simulink model "ModelEnv_Test2"  (R2020b)
settings: Solver=VariableStepAuto  StartTime=0.0  StopTime=10  RelTol=1e-3
values from neighbouring files (symbols this model uses):
  Atz = -0.15    [AgentSaboteur.m]    (also in Test1_code.m; TesterUnAgent.m; test_RL_code.m; test_RL_code_v2.m)
  Bd = 0.03    [AgentSaboteur.m]    (also in Test1_code.m; TesterUnAgent.m; test_RL_code.m; test_RL_code_v2.m)
  Bh = mdot/(3*M)    (= 0.164794600011)    [AgentSaboteur.m]    (also in Test1_code.m; TesterUnAgent.m; test_RL_code.m; test_RL_code_v2.m)
  Tout = [7 6 5 6 4 4 6 8 9 10 11 12 14 14 16 17 14 12 10 9 8 8 7 6]    [AgentSaboteur.m]    (also in Test1_code.m = out.simout.Data(:, 1); Tout(end)=[]; TesterUnAgent.m; testBlanc.m = 13 + 2*rand(1, 240); test_RL_code.m)
  Tz_init = Tout(1)    [AgentSaboteur.m]    (also in Test1_code.m; TesterUnAgent.m; testBlanc.m; test_RL_code.m)
libraries: dspsrcs4 x1
settings Model: Creator=masdoua1  LastModifiedBy=masdoua1
settings SolverCC: AlgebraicLoopSolver=LineSearch

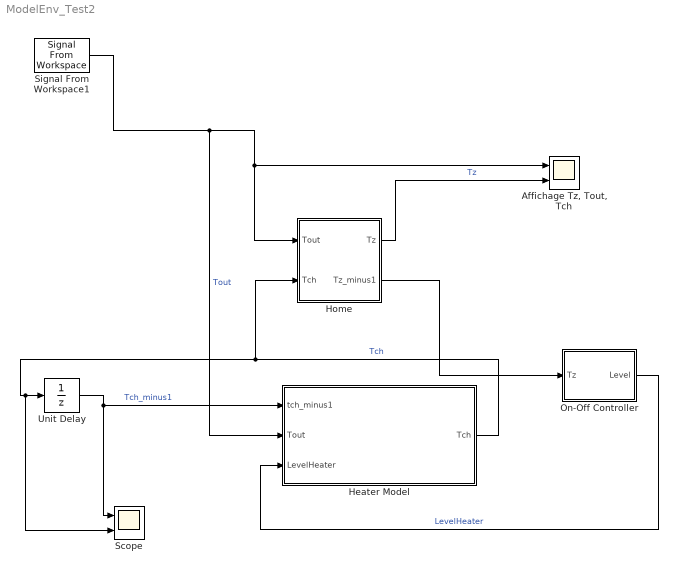
== system ModelEnv_Test2 ==
  "Affichage Tz, Tout, Tch" : Scope  NumInputPorts=2
  Heater Model : Subsystem
  Home : Subsystem
  On-Off Controller : MATLAB Function  TreatAsAtomicUnit=on
  Scope : Scope  NumInputPorts=2
  Signal From Workspace1 : dspsrcs4/Signal From Workspace  X=Tout  Ts=1  nsamps=1  OutputAfterFinalValue=Setting to zero  ignoreOrWarnInputAndFrameLengths=off  OutputFrames=off
  Unit Delay : UnitDelay  InitialCondition=Tout(1)  HasFrameUpgradeWarning=on
  wires:
  Signal From Workspace1/1 -> Heater Model/2(Tout), Home/1(Tout), "Affichage Tz, Tout, Tch"/1  "Tout"
  Home/1(Tz) -> "Affichage Tz, Tout, Tch"/2  "Tz"
  Heater Model/1(Tch) -> Scope/2, Unit Delay/1, Home/2(Tch)  "Tch"
  Unit Delay/1 -> Scope/1, Heater Model/1(tch_minus1)  "Tch_minus1"
  On-Off Controller/1(Level) -> Heater Model/3(LevelHeater)  "LevelHeater"
  Home/2(Tz_minus1) -> On-Off Controller/1(Tz)

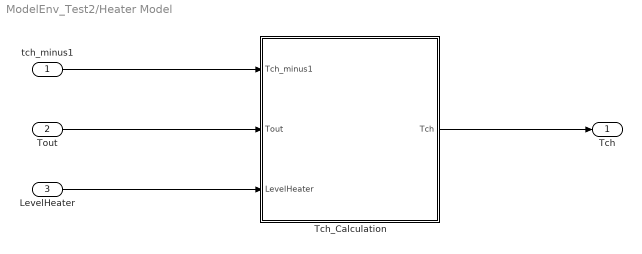
== system ModelEnv_Test2/Heater Model ==
  tch_minus1 : Inport
  Tout : Inport  Port=2
  LevelHeater : Inport  Port=3
  Tch_Calculation : MATLAB Function  TreatAsAtomicUnit=on
  Tch : Outport
  wires:
  Tout/1 -> Tch_Calculation/2(Tout)
  tch_minus1/1 -> Tch_Calculation/1(Tch_minus1)
  LevelHeater/1 -> Tch_Calculation/3(LevelHeater)
  Tch_Calculation/1(Tch) -> Tch/1

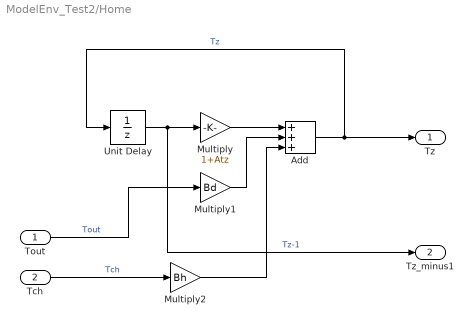
== system ModelEnv_Test2/Home ==
  Tout : Inport
  Tch : Inport  Port=2
  Add : Sum  Inputs=+++
  Multiply : Gain  Gain=1+Atz
  Multiply1 : Gain  Gain=Bd
  Multiply2 : Gain  Gain=Bh
  Unit Delay : UnitDelay  InitialCondition=Tz_init  HasFrameUpgradeWarning=on
  Tz : Outport
  Tz_minus1 : Outport  Port=2
  wires:
  Multiply/1 -> Add/1
  Unit Delay/1 -> Tz_minus1/1, Multiply/1  "Tz-1"
  Tout/1 -> Multiply1/1  "Tout"
  Multiply1/1 -> Add/2
  Add/1 -> Unit Delay/1, Tz/1  "Tz"
  Tch/1 -> Multiply2/1  "Tch"
  Multiply2/1 -> Add/3

== matlab function ModelEnv_Test2/Heater Model/Tch_Calculation ==
  data: Tch_minus1 input; Tout input; LevelHeater input; Tch output
function Tch = fcn(Tch_minus1, Tout, LevelHeater)
    
    if Tout > Tch_minus1
        Tch_minus1 = Tout; 
    end
    
    Tch = Tch_minus1 + LevelHeater;

    if LevelHeater ==0
        Tch = 0;
    end

== matlab function ModelEnv_Test2/On-Off Controller ==
  data: Tz input; Level output
function Level = fcn(Tz)

if Tz < 14
    Level =3;
else
    Level =0;
end
end
